simulink model "open_close_P_PI_PID"  (R2022b)
settings: Solver=VariableStepAuto  StartTime=0.0  StopTime=60.0  RelTol=1e-3
undefined symbols (not defined in the file): DiscIntNeverNeededParam
settings Model: Creator=yasso  LastModifiedBy=yasso

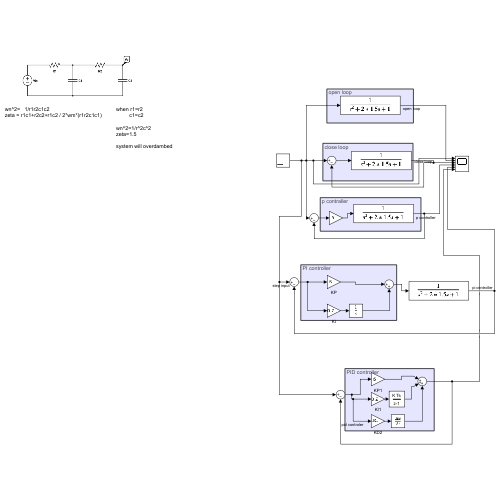
[thumbnail: Simulink's stored preview of the top-level diagram]
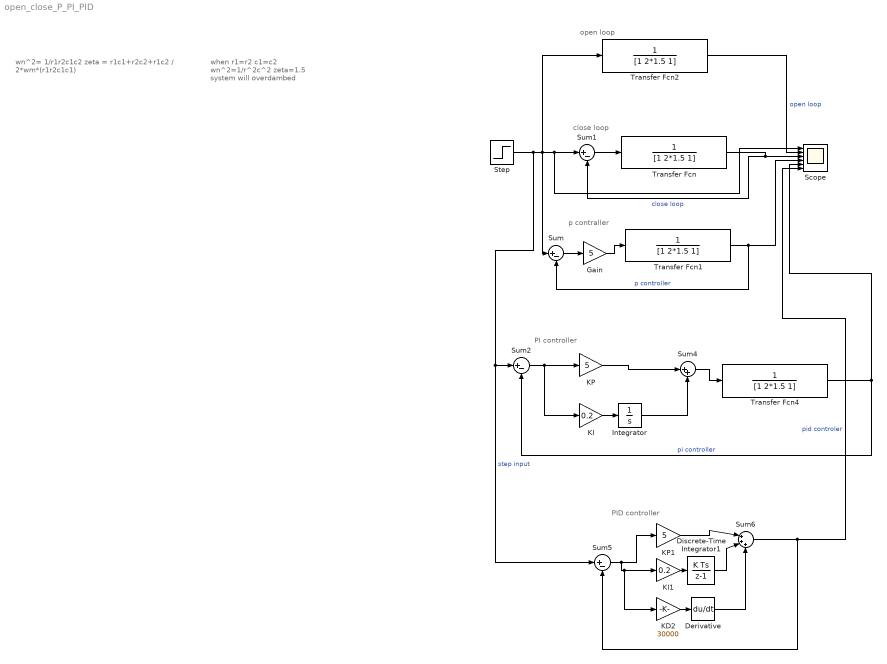
== system open_close_P_PI_PID ==
  note: open loop
  note: close loop
  note: p contraller
  note: PI controller
  note: when r1=r2
      | c1=c2
      |
      | wn^2=1/r^2c^2
      | zeta=1.5
      |
      | system will overdambed
  note: wn^2= 1/r1r2c1c2
      | zeta = r1c1+r2c2+r1c2 / 2*wm*(r1r2c1c1)
  note: PID controller
  Derivative : Derivative
  Discrete-Time Integrator1 : DiscreteIntegrator  SampleTime=-1  ICPrevOutput=DiscIntNeverNeededParam  ICPrevScaledInput=DiscIntNeverNeededParam
  Gain : Gain  Gain=5
  Integrator : Integrator
  KD2 : Gain  Gain=30000
  KI : Gain  Gain=0.2
  KI1 : Gain  Gain=0.2
  KP : Gain  Gain=5
  KP1 : Gain  Gain=5
  Scope : Scope  NumInputPorts=6
  Step : Step  SampleTime=0
  Sum{,1..2,5} (4 alike) : Sum  Inputs=|+-
  Sum4 : Sum  Inputs=|++
  Sum6 : Sum  Inputs=|+++
  Transfer Fcn{,1..2,4} (4 alike) : TransferFcn  Denominator=[1 2*1.5 1]
  wires:
  Transfer Fcn1/1 -> Scope/4, Sum/2  "p controller"
  Transfer Fcn/1 -> Sum1/2, Scope/3  "close loop"
  Sum/1 -> Gain/1
  Sum1/1 -> Transfer Fcn/1
  Gain/1 -> Transfer Fcn1/1
  Transfer Fcn2/1 -> Scope/2  "open loop"
  Sum4/1 -> Transfer Fcn4/1
  Transfer Fcn4/1 -> Scope/5, Sum2/2  "pi controller"
  Step/1 -> Sum5/1, Sum2/1, Transfer Fcn2/1, Sum/1, Sum1/1, Scope/1  "step input"
  Sum2/1 -> KI/1, KP/1
  KP/1 -> Sum4/1
  KI/1 -> Integrator/1
  Integrator/1 -> Sum4/2
  KI1/1 -> Discrete-Time Integrator1/1
  Sum6/1 -> Sum5/2, Scope/6  "pid controler"
  Discrete-Time Integrator1/1 -> Sum6/2
  KP1/1 -> Sum6/1
  Sum5/1 -> KP1/1, KD2/1, KI1/1
  KD2/1 -> Derivative/1
  Derivative/1 -> Sum6/3
